simulink model "modello_controllore"  (R2025a)
settings: Solver=ode4  StartTime=0.0  StopTime=10.0  FixedStep=Ts  RelTol=1e-3
values from neighbouring files (symbols this model uses):
  K = 500    [FUNZIONA_CHISSA.m]    (also in identificazione_diagrammi_bode.m; robot_diverse_traiettorie.m = 2000; run_robot_simulation.m = 2000)
  Kd_tau = 0.1    [robot_diverse_traiettorie.m]    (also in run_robot_simulation.m)
  Kd_theta = 20    [robot_diverse_traiettorie.m]    (also in run_robot_simulation.m = 0.5)
  Kp_tau = 10    [robot_diverse_traiettorie.m]    (also in run_robot_simulation.m)
  Kp_theta = 70    [robot_diverse_traiettorie.m]    (also in run_robot_simulation.m = 2)
  M = 2    [FUNZIONA_CHISSA.m]    (also in identificazione_diagrammi_bode.m; robot_diverse_traiettorie.m; run_robot_simulation.m)
  Mm = 0.5    [FUNZIONA_CHISSA.m]    (also in identificazione_diagrammi_bode.m; robot_diverse_traiettorie.m; run_robot_simulation.m)
settings Model: Creator=hp  LastModifiedBy=alessandrodichiara
settings DataIOCC: SaveFormat=StructureWithTime  SaveOutput=off

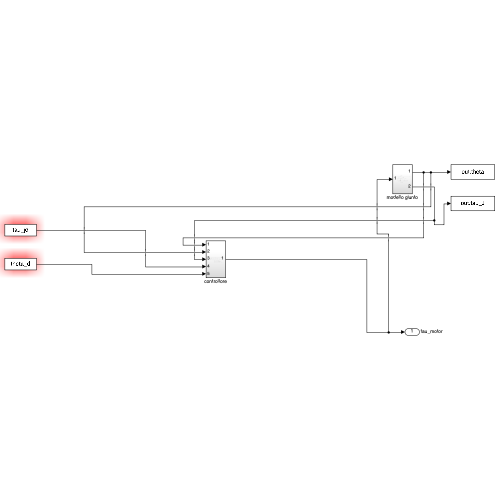
[thumbnail: Simulink's stored preview of the top-level diagram]
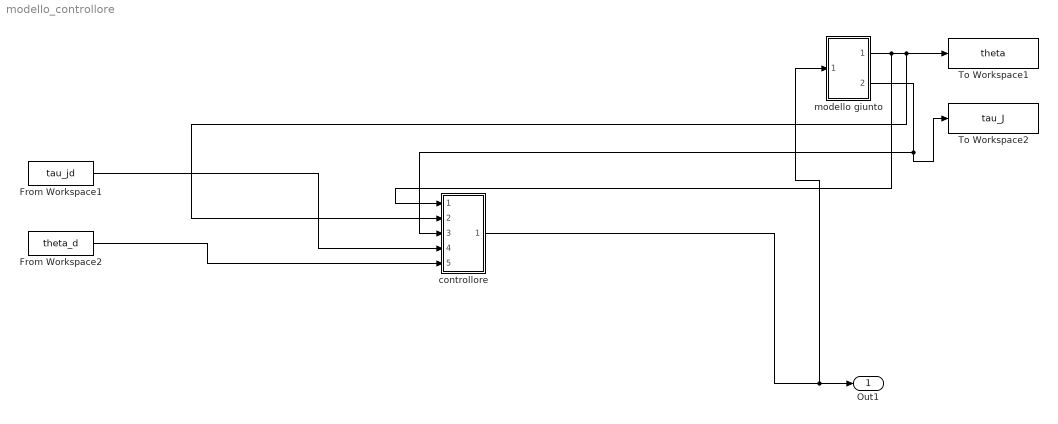
== system modello_controllore ==
  From Workspace1 : FromWorkspace  VariableName=tau_jd
  From Workspace2 : FromWorkspace  VariableName=theta_d
  To Workspace1 : ToWorkspace  VariableName=theta  SaveFormat=Timeseries  SampleTime=-1
  To Workspace2 : ToWorkspace  VariableName=tau_J  SaveFormat=Timeseries  SampleTime=-1
  controllore : Subsystem
  modello giunto : Subsystem
  Out1 : Outport  SignalName=tau_motor
  wires:
  modello giunto/1(Out1) -> controllore/1(In1), controllore/2(In2), To Workspace1/1
  modello giunto/2(Out2) -> controllore/3(In3), To Workspace2/1
  controllore/1(Out1) -> modello giunto/1(In1), Out1/1
  From Workspace1/1 -> controllore/4(In4)
  From Workspace2/1 -> controllore/5(In5)

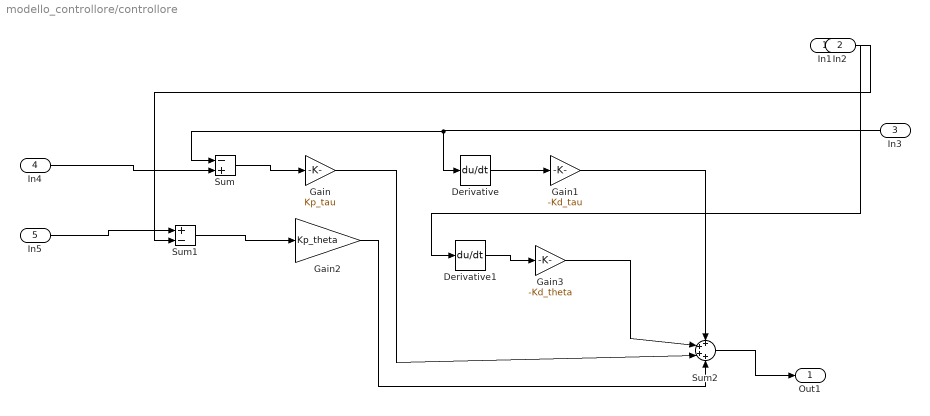
== system modello_controllore/controllore ==
  In1 : Inport
  In2 : Inport  Port=2
  In3 : Inport  Port=3
  In4 : Inport  Port=4
  In5 : Inport  Port=5
  Derivative : Derivative
  Derivative1 : Derivative
  Gain : Gain  Gain=Kp_tau
  Gain1 : Gain  Gain=-Kd_tau
  Gain2 : Gain  Gain=Kp_theta
  Gain3 : Gain  Gain=-Kd_theta
  Sum : Sum  Inputs=-+
  Sum1 : Sum  Inputs=+-
  Sum2 : Sum  Inputs=++++
  Out1 : Outport
  wires:
  In1/1 -> Derivative1/1
  In2/1 -> Sum1/2
  In5/1 -> Sum1/1
  Derivative/1 -> Gain1/1
  Sum1/1 -> Gain2/1
  Gain1/1 -> Sum2/1
  Sum/1 -> Gain/1
  In3/1 -> Derivative/1, Sum/1
  Gain2/1 -> Sum2/4
  Derivative1/1 -> Gain3/1
  Gain/1 -> Sum2/3
  Sum2/1 -> Out1/1
  In4/1 -> Sum/2
  Gain3/1 -> Sum2/2

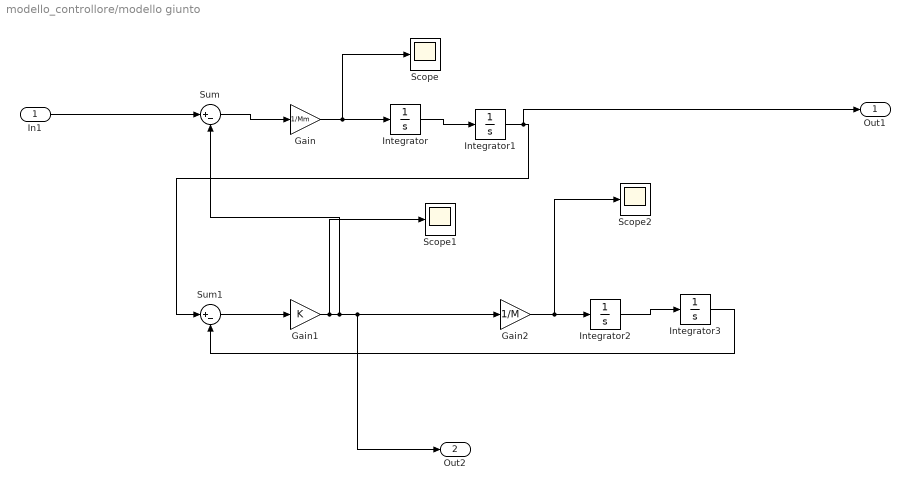
== system modello_controllore/modello giunto ==
  In1 : Inport
  Gain : Gain  Gain=1/Mm
  Gain1 : Gain  Gain=K
  Gain2 : Gain  Gain=1/M
  Integrator{,1..3} (4 alike) : Integrator
  Scope : Scope
      settings: ActiveDisplayYMinimum=-10.16007  ActiveDisplayYMaximum=9.02572
  Scope1 : Scope
      settings: ActiveDisplayYMinimum=-5.65054  ActiveDisplayYMaximum=6.14623
  Scope2 : Scope
      settings: ActiveDisplayYMinimum=-3.76702  ActiveDisplayYMaximum=4.09748  DataLoggingVariableName=ScopeData2
  Sum : Sum  Inputs=|+-
  Sum1 : Sum  Inputs=|+-
  Out1 : Outport
  Out2 : Outport  Port=2
  wires:
  In1/1 -> Sum/1
  Gain/1 -> Scope/1, Integrator/1
  Integrator2/1 -> Integrator3/1
  Sum/1 -> Gain/1
  Integrator1/1 -> Out1/1, Sum1/1
  Integrator3/1 -> Sum1/2
  Sum1/1 -> Gain1/1
  Integrator/1 -> Integrator1/1
  Gain1/1 -> Scope1/1, Sum/2, Out2/1, Gain2/1
  Gain2/1 -> Scope2/1, Integrator2/1
